simulink model "SimulationIA"  (R2022a)
settings: Solver=ode45  StartTime=0.0  StopTime=20  MaxStep=0.1  RelTol=1e-6  EnableMultiTasking=on
undefined symbols (not defined in the file or in its folder): Balanduino, DiscIntNeverNeededParam, Kaug
settings Model: Creator=studio  LastModifiedBy=ja125
settings SolverCC: AlgebraicLoopSolver=TrustRegion
settings DataIOCC: LimitDataPoints=on  SaveFormat=Array  SignalLoggingSaveFormat=ModelDataLogs  ReturnWorkspaceOutputs=off
settings OptimizationCC: ExpressionDepthLimit=2147483647  LifeSpan=inf
settings DebuggingCC: UnderspecifiedInitializationDetection=Classic  MergeDetectMultiDrivingBlocksExec=none  SolverPrmCheckMsg=warning  FcnCallInpInsideContextMsg=warning  UnconnectedInputMsg=warning  UnconnectedOutputMsg=warning  UnconnectedLineMsg=warning  StateNameClashWarn=warning  SFUnexpectedBacktrackingDiag=warning  SFNoUnconditionalDefaultTransitionDiag=warning  SFExecutionAtInitializationDiag=none  SFMachineParentedDataDiag=warning  ArithmeticOperatorsInVariantConditions=warning
settings HardwareCC: ProdBitPerPointer=32  ProdBitPerSizeT=32  ProdBitPerPtrDiffT=32  ProdLargestAtomicFloat=None  ProdIntDivRoundTo=Undefined  ProdEndianess=Unspecified  ProdWordSize=32  ProdHWDeviceType=32-bit Generic
settings ModelReferenceCC: PropagateSignalLabelsOutOfModel=off
settings SFSimCC: SimUseLocalCustomCode=off  CustomCodeUndefinedFunction=UseInterfaceOnly
settings RTWCC: RTWUseLocalCustomCode=off
settings CodeAppCC: StateflowObjectComments=on
settings GRTTargetCC: TargetLangStandard=C89/C90 (ANSI)
settings ConfigComp: CovMetricSettings=dw  CovSaveCumulativeToWorkspaceVar=on  CovSaveSingleToWorkspaceVar=on  CovExternalEMLEnable=off

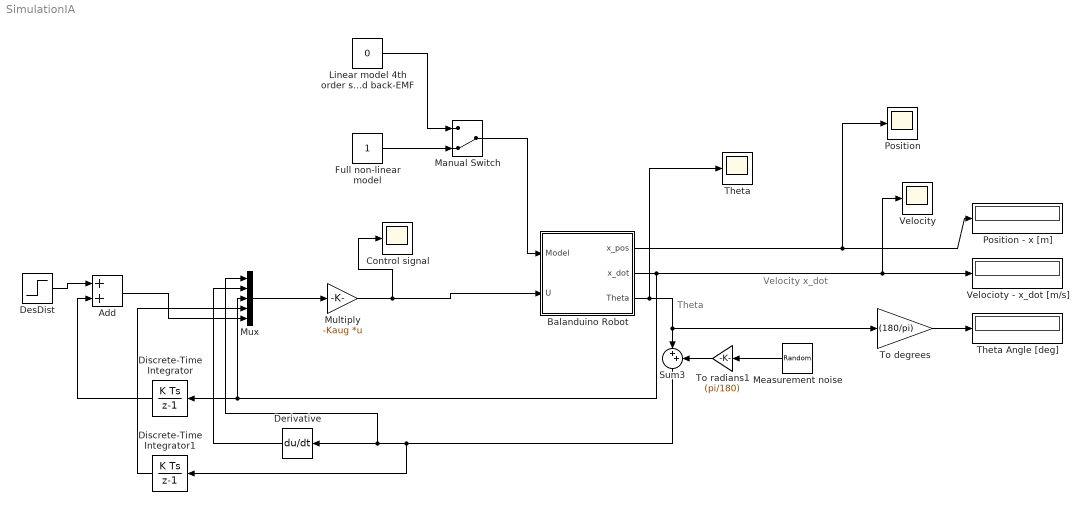
== system SimulationIA ==
  note: Theta
  note: Velocity
      | x_dot
  Add : Sum
  Balanduino Robot : Subsystem  mask(Inverted pendulum on cart){Mb=Balanduino.M, m=Balanduino.m, d=Balanduino.d, r=Balanduino.r, Ra=Balanduino.Ra, La=Balanduino.La, Km=Balanduino.Km, Ku=Balanduino.Ku, g=Balanduino.g}
      mask prompts: Mb "Mass of main body"; m "Mass of battery"; d "Distance whell axis - battery"; r "Wheel radius"; Ra "Motor resistance"; La "Motor inductance"; Km "Motor current-torque"; Ku "Motor back-emf"; g "Acceleration of gravity"
      mask help: Unmask and double-click to see dynamics
      mask Help: Nonlinear dynamics of inverted pendulum on cart.
  Control signal : Scope
  Derivative : Derivative
  DesDist : Step  After=0  SampleTime=0
  Discrete-Time Integrator : DiscreteIntegrator  SampleTime=-1  ICPrevOutput=DiscIntNeverNeededParam  ICPrevScaledInput=DiscIntNeverNeededParam
  Discrete-Time Integrator1 : DiscreteIntegrator  SampleTime=-1  ICPrevOutput=DiscIntNeverNeededParam  ICPrevScaledInput=DiscIntNeverNeededParam
  Full non-linear model : Constant
  Linear model 4th order system with motor inductance and back-EMF : Constant  Value=0
  Manual Switch : ManualSwitch  CurrentSetting=0
  Measurement noise : RandomNumber  Variance=5  Seed=1337  SampleTime=0.1
  Multiply : Gain  Gain=-Kaug  Multiplication=Matrix(K*u)
  Mux : Mux  Inputs=5
  Position : Scope
  Position - x [m] : Display
  Sum3 : Sum  Inputs=|++
  Theta : Scope
  Theta Angle [deg] : Display
  To degrees : Gain  Gain=(180/pi)
  To radians1 : Gain  Gain=(pi/180)
  Velocioty - x_dot [m/s] : Display
  Velocity : Scope
  wires:
  Linear model 4th order system with motor inductance and back-EMF/1 -> Manual Switch/1
  Full non-linear model/1 -> Manual Switch/2
  Manual Switch/1 -> Balanduino Robot/1(Model)
  Balanduino Robot/2(x_dot) -> Velocioty - x_dot [m/s]/1, Velocity/1, Mux/3, Discrete-Time Integrator/1
  Balanduino Robot/3(Theta) -> Theta/1, Sum3/1, To degrees/1
  To degrees/1 -> Theta Angle [deg]/1
  To radians1/1 -> Sum3/2
  Balanduino Robot/1(x_pos) -> Position - x [m]/1, Position/1
  Measurement noise/1 -> To radians1/1
  Multiply/1 -> Control signal/1, Balanduino Robot/2(U)
  Mux/1 -> Multiply/1
  DesDist/1 -> Add/1
  Discrete-Time Integrator/1 -> Add/2
  Sum3/1 -> Discrete-Time Integrator1/1, Mux/1, Derivative/1
  Derivative/1 -> Mux/2
  Add/1 -> Mux/5
  Discrete-Time Integrator1/1 -> Mux/4

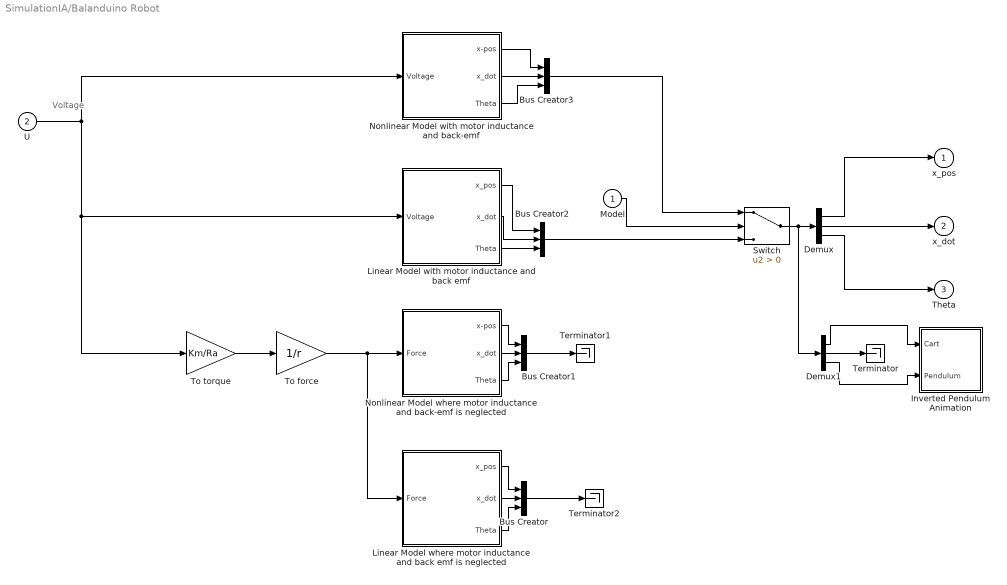
== system SimulationIA/Balanduino Robot ==
  note: Voltage
  Model : Inport
  U : Inport  Port=2
  Bus Creator{,1..3} (4 alike) : BusCreator  Inputs=3
  Demux : Demux  Outputs=3
  Demux1 : Demux  Outputs=3
  Inverted Pendulum Animation : Subsystem
  Linear Model where motor inductance and back emf is neglected : Subsystem
  "Linear Model with motor inductance and back emf " : Subsystem
  Nonlinear Model with motor inductance and back-emf : Subsystem
  Nonlinear Model where motor inductance and back-emf is neglected : Subsystem
  Switch : Switch  Criteria=u2 > Threshold  SaturateOnIntegerOverflow=off  InputSameDT=off
  Terminator : Terminator
  Terminator1 : Terminator
  Terminator2 : Terminator
  To force : Gain  Gain=1/r
  To torque : Gain  Gain=Km/Ra
  x_pos : Outport  InitialOutput=0
  x_dot : Outport  Port=2  InitialOutput=0
  Theta : Outport  Port=3  InitialOutput=0
  wires:
  Bus Creator/1 -> Terminator2/1
  Bus Creator1/1 -> Terminator1/1
  Bus Creator2/1 -> Switch/3
  "Linear Model with motor inductance and back emf "/3(Theta) -> Bus Creator2/3
  "Linear Model with motor inductance and back emf "/2(x_dot) -> Bus Creator2/2
  "Linear Model with motor inductance and back emf "/1(x_pos) -> Bus Creator2/1
  Bus Creator3/1 -> Switch/1
  Nonlinear Model with motor inductance and back-emf/3(Theta) -> Bus Creator3/3
  Nonlinear Model with motor inductance and back-emf/1(x-pos) -> Bus Creator3/1
  Nonlinear Model with motor inductance and back-emf/2(x_dot) -> Bus Creator3/2
  U/1 -> To torque/1, "Linear Model with motor inductance and back emf "/1(Voltage), Nonlinear Model with motor inductance and back-emf/1(Voltage)
  Demux1/2 -> Terminator/1
  Demux1/3 -> Inverted Pendulum Animation/2(Pendulum)
  Demux1/1 -> Inverted Pendulum Animation/1(Cart)
  Demux/3 -> Theta/1
  Demux/2 -> x_dot/1
  Linear Model where motor inductance and back emf is neglected/3(Theta) -> Bus Creator/3
  Linear Model where motor inductance and back emf is neglected/1(x_pos) -> Bus Creator/1
  Linear Model where motor inductance and back emf is neglected/2(x_dot) -> Bus Creator/2
  Nonlinear Model where motor inductance and back-emf is neglected/3(Theta) -> Bus Creator1/3
  Nonlinear Model where motor inductance and back-emf is neglected/2(x_dot) -> Bus Creator1/2
  Nonlinear Model where motor inductance and back-emf is neglected/1(x-pos) -> Bus Creator1/1
  Demux/1 -> x_pos/1
  Switch/1 -> Demux1/1, Demux/1
  Model/1 -> Switch/2
  To torque/1 -> To force/1
  To force/1 -> Linear Model where motor inductance and back emf is neglected/1(Force), Nonlinear Model where motor inductance and back-emf is neglected/1(Force)

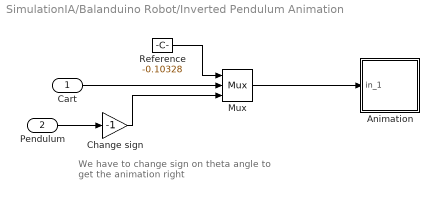
== system SimulationIA/Balanduino Robot/Inverted Pendulum Animation ==
  note: We have to change sign on theta angle
      | to get the animation right
  Cart : Inport
  Pendulum : Inport  Port=2
  Animation : Subsystem  mask(Pendulum plot){RefBlock=Reference}
      mask prompts: RefBlock "DC reference signal block name:"
      mask help: Pendulum plot
      mask Help: Pendulum animation function using Handle graphics.
      mask Display: plot([-10 10],[0 0],[-2 -2 2 2],[0 1 1 0],[0 3],[1 5])
  Change sign : Gain  Gain=-1
  Mux : Mux  Inputs=3
  Reference : Constant  Value=-0.10328
  wires:
  Reference/1 -> Mux/1
  Change sign/1 -> Mux/3
  Pendulum/1 -> Change sign/1
  Cart/1 -> Mux/2
  Mux/1 -> Animation/1(in_1)

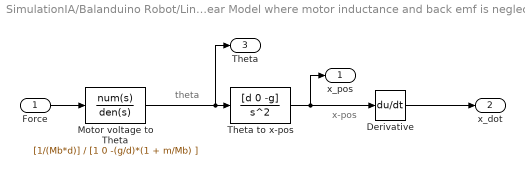
== system SimulationIA/Balanduino Robot/Linear Model where motor inductance and back emf is neglected ==
  note: x-pos
  note: theta
  Force : Inport
  Derivative : Derivative
  Motor voltage to Theta : TransferFcn  Numerator=[1/(Mb*d)]  Denominator=[1 0 -(g/d)*(1 + m/Mb) ]
  Theta to x-pos : TransferFcn  Numerator=[d 0 -g]  Denominator=[1 0 0]
  x_pos : Outport
  x_dot : Outport  Port=2
  Theta : Outport  Port=3
  wires:
  Derivative/1 -> x_dot/1
  Force/1 -> Motor voltage to Theta/1
  Theta to x-pos/1 -> Derivative/1, x_pos/1
  Motor voltage to Theta/1 -> Theta/1, Theta to x-pos/1

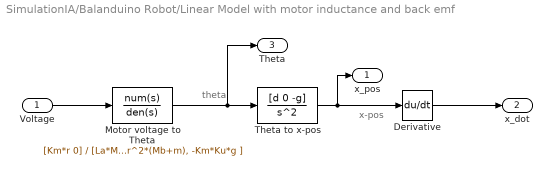
== system SimulationIA/Balanduino Robot/Linear Model with motor inductance and back emf  ==
  note: theta
  note: x-pos
  Voltage : Inport
  Derivative : Derivative
  Motor voltage to Theta : TransferFcn  Numerator=[Km*r 0]  Denominator=[La*Mb*d*r^2, Mb*Ra*d*r^2, -(La*g*r^2*(m+Mb) -Km*Ku*d ), -Ra*g*r^2*(Mb+m), -Km*Ku*g ]
  Theta to x-pos : TransferFcn  Numerator=[d 0 -g]  Denominator=[1 0 0]
  x_pos : Outport
  x_dot : Outport  Port=2
  Theta : Outport  Port=3
  wires:
  Motor voltage to Theta/1 -> Theta/1, Theta to x-pos/1
  Theta to x-pos/1 -> Derivative/1, x_pos/1
  Voltage/1 -> Motor voltage to Theta/1
  Derivative/1 -> x_dot/1

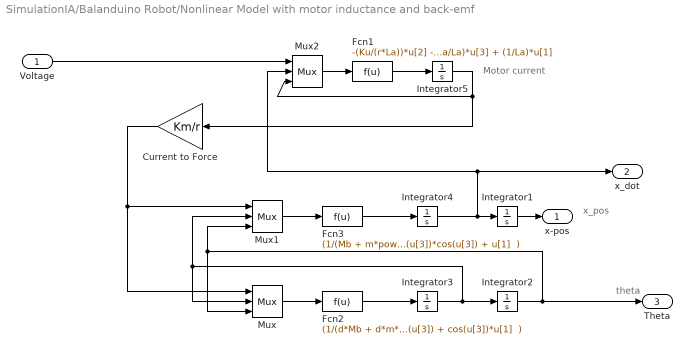
== system SimulationIA/Balanduino Robot/Nonlinear Model with motor inductance and back-emf ==
  note: Motor current
  note: theta
  note: x_pos
  Voltage : Inport
  Current to Force : Gain  Gain=Km/r
  Fcn1 : Fcn  Expr=-(Ku/(r*La))*u[2] - (Ra/La)*u[3] + (1/La)*u[1]
  Fcn2 : Fcn  Expr="(1/(d*Mb + d*m*power(sin(u[3]),2)))*( -m*d*sin(u[3])*cos(u[3])*power(u[2],2) + g*(m+Mb)*sin(u[3]) + cos(u[3])*u[1]  )"
  Fcn3 : Fcn  Expr="(1/(Mb + m*power(sin(u[3]),2)))*( -m*d*sin(u[3])*power(u[2],2) + g*m*sin(u[3])*cos(u[3]) + u[1]  )"
  Integrator{1..5} (5 alike) : Integrator
  Mux : Mux  Inputs=3
  Mux1 : Mux  Inputs=3
  Mux2 : Mux  Inputs=3
  x-pos : Outport
  x_dot : Outport  Port=2
  Theta : Outport  Port=3
  wires:
  Current to Force/1 -> Mux/1, Mux1/1
  Voltage/1 -> Mux2/1
  Integrator5/1 -> Current to Force/1, Mux2/3
  Fcn1/1 -> Integrator5/1
  Mux2/1 -> Fcn1/1
  Integrator1/1 -> x-pos/1
  Integrator2/1 -> Theta/1, Mux/3, Mux1/3
  Integrator3/1 -> Mux/2, Mux1/2, Integrator2/1
  Integrator4/1 -> x_dot/1, Mux2/2, Integrator1/1
  Fcn3/1 -> Integrator4/1
  Mux1/1 -> Fcn3/1
  Mux/1 -> Fcn2/1
  Fcn2/1 -> Integrator3/1

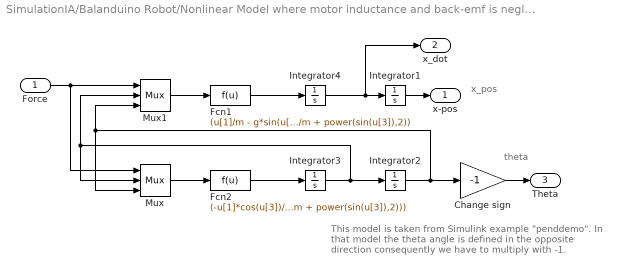
== system SimulationIA/Balanduino Robot/Nonlinear Model where motor inductance and back-emf is neglected ==
  note: This model is taken from Simulink example "penddemo".
      | In that model the theta angle is defined in the opposite
      | direction consequently we have to multiply with -1.
  note: theta
  note: x_pos
  Force : Inport
  Change sign : Gain  Gain=-1
  Fcn1 : Fcn  Expr=(u[1]/m - g*sin(u[3])*cos(u[3]) + d*power(u[2],2)*sin(u[3]))/(Mb/m + power(sin(u[3]),2))
  Fcn2 : Fcn  Expr=(-u[1]*cos(u[3])/m + (Mb+m)*g*sin(u[3])/m - d*power(u[2],2)*sin(u[3])*cos(u[3]))/(d*(Mb/m + power(sin(u[3]),2)))
  Integrator{1..4} (4 alike) : Integrator
  Mux : Mux  Inputs=3
  Mux1 : Mux  Inputs=3
  x-pos : Outport
  x_dot : Outport  Port=2
  Theta : Outport  Port=3
  wires:
  Change sign/1 -> Theta/1
  Integrator1/1 -> x-pos/1
  Force/1 -> Mux/1, Mux1/1
  Integrator2/1 -> Change sign/1, Mux/3, Mux1/3
  Integrator3/1 -> Mux/2, Mux1/2, Integrator2/1
  Integrator4/1 -> x_dot/1, Integrator1/1
  Fcn1/1 -> Integrator4/1
  Mux1/1 -> Fcn1/1
  Mux/1 -> Fcn2/1
  Fcn2/1 -> Integrator3/1

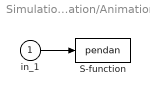
== system SimulationIA/Balanduino Robot/Inverted Pendulum Animation/Animation ==
  in_1 : Inport
  S-function : S-Function  FunctionName=pendan  Parameters=RefBlock  SFunctionDeploymentMode=off  EnableBusSupport=off
      settings: DeleteFcn=pendan([],[],[],'DeleteBlock');
  wires:
  in_1/1 -> S-function/1
